simulink model "state_space"  (R2024b)
settings: Solver=ode1  StartTime=0.0  StopTime=inf  FixedStep=dt  MaxStep=1/30  RelTol=1e-3
undefined symbols (not defined in the file or in its folder): f, G, K, Kb, Ki, Kx, y0
libraries: simulink x5, instrumentlib x2
settings Model: Creator=aalessan  LastModifiedBy=aalessan

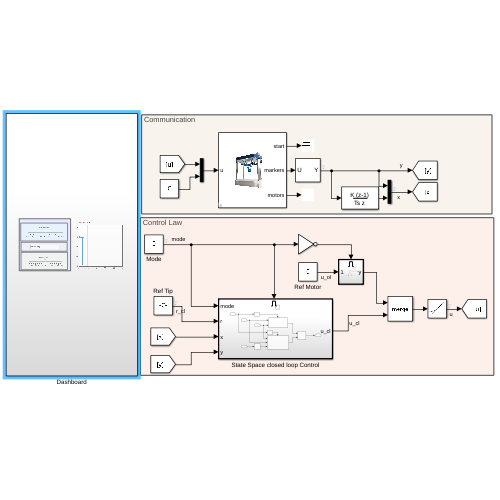
[thumbnail: Simulink's stored preview of the top-level diagram]
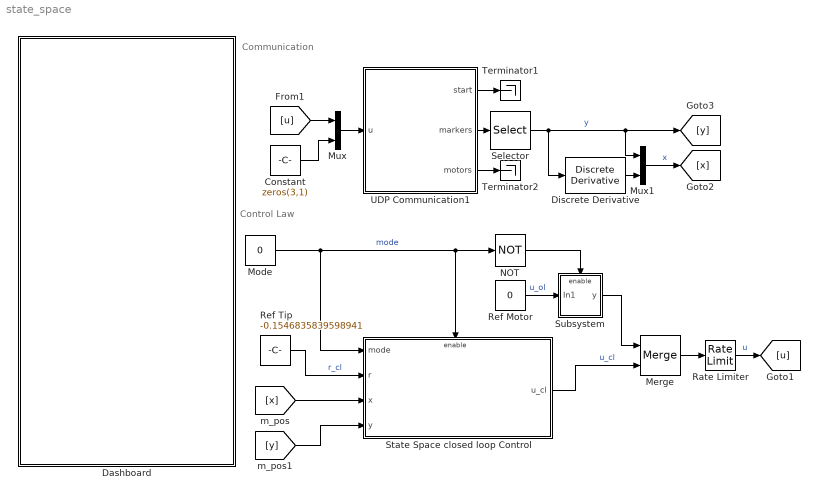
== system state_space ==
  note: Control Law
  note: Communication
  Constant : Constant  Value=zeros(3,1)
  Dashboard : Subsystem
  Discrete Derivative : simulink/Discrete/Discrete Derivative  gainval=1.0  ICPrevScaledInput=0.0  OutMin=[]  OutMax=[]  OutDataType=fixdt(1, 16)  OutScaling=2^-10  DoSatur=off
  Merge : Merge  InitialOutput=zeros(1,1)
  Mode : Constant  Value=0
  Mux : Mux  Inputs=2
  Mux1 : Mux  Inputs=2
  NOT : Logic  Operator=NOT  IconShape=distinctive  AllPortsSameDT=off  OutDataTypeStr=boolean
  Rate Limiter : RateLimiter  RisingSlewLimit=7.906  FallingSlewLimit=-7.906  SampleTimeMode=inherited
  Ref Motor : Constant  Value=0
  Ref Tip : Constant  Value=-0.1546835839598941
  Selector : Selector  InputPortWidth=6  IndexOptions=Index vector (dialog)  Indices=[3 6]  OutputSizes=1
  State Space closed loop Control : Subsystem
  Subsystem : Subsystem
  Terminator1 : Terminator
  Terminator2 : Terminator
  UDP Communication1 : Subsystem  mask{nb_markers=2, markers_init=y0}
      mask prompts: nb_markers "Nb Markers"; markers_init "Initial Markers Position"
      mask Display: image('emio.png', [0,0,10,0,50,50]);
  wires:
  Ref Tip/1 -> State Space closed loop Control/2(r)  "r_cl"
  NOT/1 -> Subsystem/Enable
  Rate Limiter/1 -> [u]  "u"
  Ref Motor/1 -> Subsystem/1(In1)  "u_ol"
  [x] -> State Space closed loop Control/3(x)
  Mode/1 -> NOT/1, State Space closed loop Control/Enable, State Space closed loop Control/1(mode)  "mode"
  Merge/1 -> Rate Limiter/1
  Subsystem/1(y) -> Merge/1
  State Space closed loop Control/1(u_cl) -> Merge/2  "u_cl"
  [y] -> State Space closed loop Control/4(y)
  UDP Communication1/1(start) -> Terminator1/1
  UDP Communication1/3(motors) -> Terminator2/1
  Mux/1 -> UDP Communication1/1(u)
  Constant/1 -> Mux/2
  Selector/1 -> Discrete Derivative/1, Mux1/1, [y]  "y"
  [u] -> Mux/1
  UDP Communication1/2(markers) -> Selector/1
  Discrete Derivative/1 -> Mux1/2
  Mux1/1 -> [x]  "x"

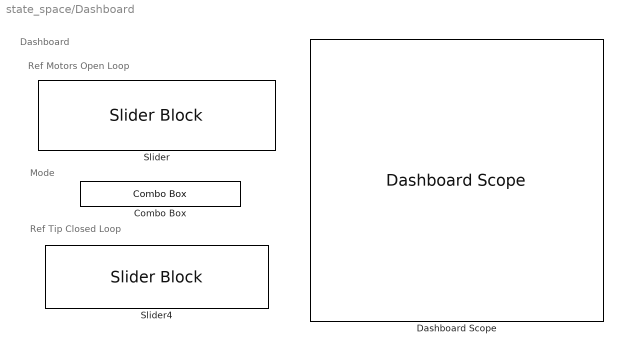
== system state_space/Dashboard ==
  note: Mode
  note: Ref Tip Closed Loop
  note: Dashboard
  note: Ref Motors Open Loop
  Combo Box : ComboBox  LabelPosition=Hide  SelectedLabel=Open Loop
      settings: Values={{'Open Loop', 'State Feedback', 'State Feedback Integral'}, [0 1 2]}
  Dashboard Scope : DashboardScope  Ymin=-50  Ymax=50  UpdateMode=Scroll
  Slider : SliderBlock  ScaleMin=-1.57  ScaleMax=1.57
  Slider4 : SliderBlock  ScaleMin=-50  ScaleMax=50

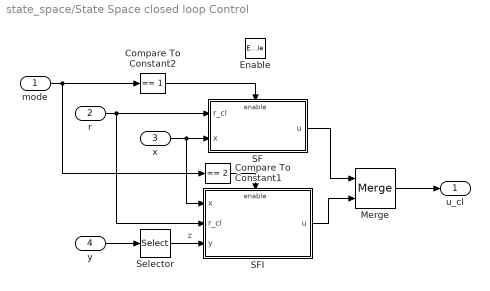
== system state_space/State Space closed loop Control ==
  mode : Inport
  r : Inport  Port=2
  x : Inport  Port=3
  y : Inport  Port=4
  Enable : EnablePort  StatesWhenEnabling=reset
  Compare To Constant1 : simulink/Logic and Bit Operations/Compare To Constant  relop===  const=2  OutDataTypeStr=boolean
  Compare To Constant2 : simulink/Logic and Bit Operations/Compare To Constant  relop===  const=1  OutDataTypeStr=boolean
  Merge : Merge
  SF : Subsystem
  SFI : Subsystem
  Selector : Selector  InputPortWidth=2  IndexOptions=Index vector (dialog)  Indices=[1]  OutputSizes=1
  u_cl : Outport
  wires:
  r/1 -> SFI/2(r_cl), SF/1(r_cl)
  Merge/1 -> u_cl/1
  y/1 -> Selector/1
  x/1 -> SFI/1(x), SF/2(x)
  Selector/1 -> SFI/3(y)  "z"
  SFI/1(u) -> Merge/2
  SF/1(u) -> Merge/1
  mode/1 -> Compare To Constant2/1, Compare To Constant1/1
  Compare To Constant2/1 -> SF/Enable
  Compare To Constant1/1 -> SFI/Enable

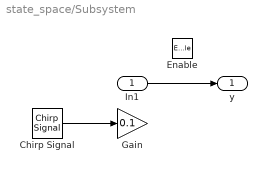
== system state_space/Subsystem ==
  In1 : Inport
  Enable : EnablePort
  Chirp Signal : simulink/Sources/Chirp Signal  f1=0.05  T=10  f2=2
  Gain : Gain  Gain=0.1
  y : Outport
  wires:
  Chirp Signal/1 -> Gain/1
  In1/1 -> y/1

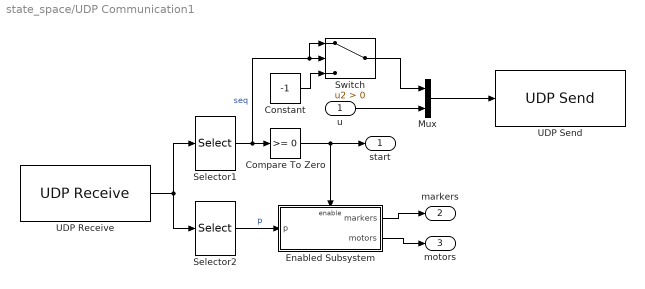
== system state_space/UDP Communication1 ==
  u : Inport
  Compare To Zero : simulink/Logic and Bit Operations/Compare To Zero  relop=>=  OutDataTypeStr=boolean
  Constant : Constant  Value=-1
  Enabled Subsystem : Subsystem  TreatAsAtomicUnit=on
  Mux : Mux  Inputs=2
  Selector1 : Selector  InputPortWidth=5+3*nb_markers  IndexOptions=Index vector (dialog)  Indices=[1]  OutputSizes=1
  Selector2 : Selector  InputPortWidth=5+3*nb_markers  IndexOptions=Index vector (dialog)  Indices=2:5+3*nb_markers  OutputSizes=1
  Switch : Switch  Criteria=u2 > Threshold  SaturateOnIntegerOverflow=off  InputSameDT=off
  UDP Receive : instrumentlib/UDP Receive  LocalAddress=127.0.0.1  LocalPort=25000  EnablePortSharing=off  Host=127.0.0.1  Port=9090  GetLatestData=on  DataSize=[ 3*nb_markers+5, 1 ]  DataType=double  ASCIIFormatting=%f,  Terminator=LF  CustomTerminator=10  ByteOrder=little-endian  EnableBlockingMode=on  Timeout=0.1  SampleTime=-1  SimulateUsing=Interpreted execution
  UDP Send : instrumentlib/UDP Send  Host=127.0.0.1  Port=25001  LocalAddress=0.0.0.0  LocalPort=-1  EnablePortSharing=off  OutputDatagramPacketSize=512  ByteOrder=little-endian  EnableBlockingMode=on  SimulateUsing=Interpreted execution
  start : Outport
  markers : Outport  Port=2
  motors : Outport  Port=3
  wires:
  Mux/1 -> UDP Send/1
  u/1 -> Mux/2
  Enabled Subsystem/2(motors) -> motors/1
  Selector2/1 -> Enabled Subsystem/1(p)  "p"
  Enabled Subsystem/1(markers) -> markers/1
  Selector1/1 -> Switch/1, Switch/2, Compare To Zero/1  "seq"
  Compare To Zero/1 -> start/1, Enabled Subsystem/Enable
  Constant/1 -> Switch/3
  UDP Receive/1 -> Selector1/1, Selector2/1
  Switch/1 -> Mux/1

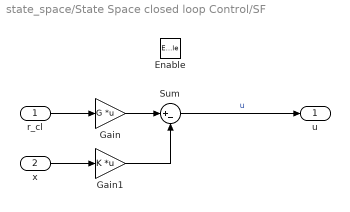
== system state_space/State Space closed loop Control/SF ==
  r_cl : Inport
  x : Inport  Port=2
  Enable : EnablePort  StatesWhenEnabling=reset
  Gain : Gain  Gain=G  Multiplication=Matrix(K*u)
  Gain1 : Gain  Gain=K  Multiplication=Matrix(K*u)
  Sum : Sum  Inputs=|+-
  u : Outport
  wires:
  Gain1/1 -> Sum/2
  Gain/1 -> Sum/1
  Sum/1 -> u/1  "u"
  r_cl/1 -> Gain/1
  x/1 -> Gain1/1

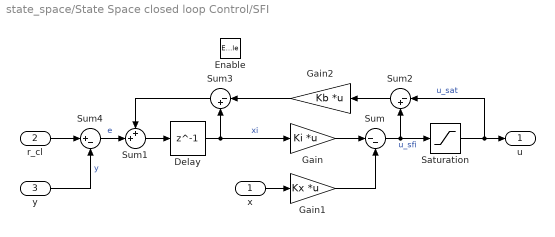
== system state_space/State Space closed loop Control/SFI ==
  x : Inport
  r_cl : Inport  Port=2
  y : Inport  Port=3
  Enable : EnablePort  StatesWhenEnabling=reset
  Delay : Delay  DelayLength=1
  Gain : Gain  Gain=Ki  Multiplication=Matrix(K*u)
  Gain1 : Gain  Gain=Kx  Multiplication=Matrix(K*u)
  Gain2 : Gain  Gain=Kb  Multiplication=Matrix(K*u)
  Saturation : Saturate  UpperLimit=1.57  LowerLimit=-1.57
  Sum : Sum  Inputs=|--
  Sum1 : Sum  Inputs=++|
  Sum2 : Sum  Inputs=|-+
  Sum3 : Sum  Inputs=|-+
  Sum4 : Sum  Inputs=|+-
  u : Outport
  wires:
  Gain1/1 -> Sum/2
  Gain/1 -> Sum/1
  Saturation/1 -> Sum2/1, u/1  "u_sat"
  x/1 -> Gain1/1
  Sum1/1 -> Delay/1
  y/1 -> Sum4/2  "y"
  r_cl/1 -> Sum4/1
  Delay/1 -> Sum3/2, Gain/1  "xi"
  Sum/1 -> Sum2/2, Saturation/1  "u_sfi"
  Sum2/1 -> Gain2/1
  Sum3/1 -> Sum1/1
  Sum4/1 -> Sum1/2  "e"
  Gain2/1 -> Sum3/1

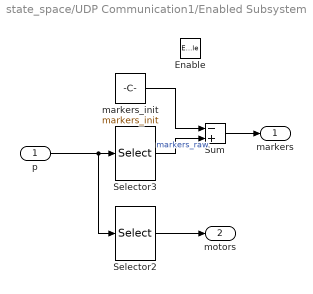
== system state_space/UDP Communication1/Enabled Subsystem ==
  p : Inport
  Enable : EnablePort
  Selector2 : Selector  InputPortWidth=4+3*nb_markers  IndexOptions=Index vector (dialog)  Indices=3*nb_markers+1:4+3*nb_markers  OutputSizes=1
  Selector3 : Selector  InputPortWidth=4+3*nb_markers  IndexOptions=Index vector (dialog)  Indices=1:3*nb_markers  OutputSizes=1
  Sum : Sum  Inputs=-+
  markers_init : Constant  Value=markers_init
  markers : Outport
  motors : Outport  Port=2
  wires:
  Sum/1 -> markers/1
  p/1 -> Selector2/1, Selector3/1
  Selector2/1 -> motors/1
  markers_init/1 -> Sum/1
  Selector3/1 -> Sum/2  "markers_raw"
